simulink model "transfer_function_calculation"  (R2016a)
settings: Solver=VariableStepAuto  StartTime=0.0  StopTime=5  RelTol=1e-3
values from neighbouring files (symbols this model uses):
  a = .7    (= 0.7)    [PM_1_5MW_syn_27.m]
  Flux = 5.8264    [PM_1_5MW_syn_27.m]
  Id_set = 500    [PM_1_5MW_syn_27.m]
  Iq_set = -2200    [PM_1_5MW_syn_27.m]
  L = .0001    (= 0.0001)    [PM_1_5MW_syn_27.m]
  Ld = 0.001575    [PM_1_5MW_syn_27.m]
  Lq = 0.001575    [PM_1_5MW_syn_27.m]
  mn = 60000    [PM_1_5MW_syn_27.m]
  p = 26    [PM_1_5MW_syn_27.m]
  Rs = 0.000821    [PM_1_5MW_syn_27.m]
  Sollkurve_M_Optimum = [0 57121 101549 158670 228485 310994 406196 514092 634681 767965 810425 823386 ... (13 elements, 13x1)]    [Lookup_M_n.mat]
  Sollkurve_nGen_Optimum = [0 5 7 9 11 12 14 16 18 20 20.07 20.2 ... (13 elements, 13x1)]    [Lookup_M_n.mat]
  Speed_set = w_m    (= 2.10172548525)    [PM_1_5MW_syn_27.m]
  Ts_Power = 5.000000000000000e-06    (= 5e-06)    [PM_1_5MW_syn_27.m]
  Vdc = 1200    [PM_1_5MW_syn_27.m]
  Vh = Vm/6*0    (= 0)    [PM_1_5MW_syn_27.m]
undefined symbols (not defined in the file or in its folder): C2, Esw_Erec, Esw_Off, Esw_On, Page_Temp_C
undefined symbols (not defined in the file): Ts_Control, z
libraries: fl_lib x84, powerlib_meascontrol x58, simulink x56, nesl_utility x36, powerlib x33, simulink_extras x11
(part 6 of 6)

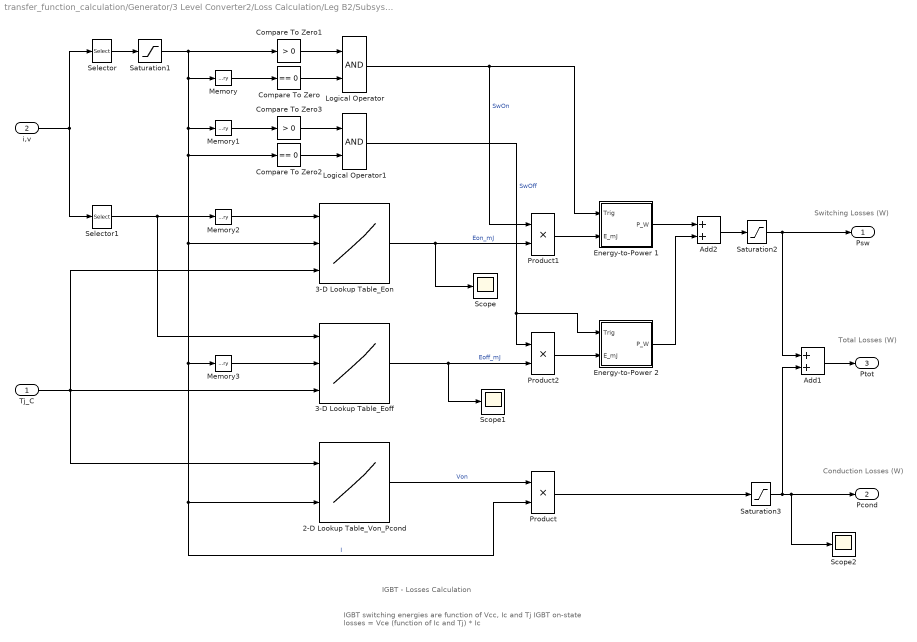
== system transfer_function_calculation/Generator/3 Level Converter2/Loss Calculation/Leg B2/Subsystem/Loss Calculation Unit/IGBTs Losses Calculation ==
  note: IGBT - Losses Calculation
  note: Switching Losses (W)
  note: Conduction Losses (W)
  note: Total Losses (W)
  note: IGBT switching energies are function of Vcc, Ic and Tj
      | IGBT on-state losses = Vce (function of Ic and Tj) * Ic
  Tj_C : Inport
  i,v : Inport  Port=2  PortDimensions=4
  2-D Lookup Table_Von_Pcond : Lookup_n-D  BreakpointsForDimension1=IGBT_Tj_OnState  BreakpointsForDimension2=IGBT_Ic_OnState  BreakpointsForDimension3=Page_Temp_C  Table=IGBT_Vce_OnState  RndMeth=Simplest  InputSameDT=on
  3-D Lookup Table_Eoff : Lookup_n-D  NumberOfTableDimensions=3  BreakpointsForDimension1=Vcc_Esw_Off  BreakpointsForDimension2=IGBT_Ic_Eoff  BreakpointsForDimension3=IGBT_Tj_Eoff  Table=Esw_Off  RndMeth=Simplest  InputSameDT=on
  3-D Lookup Table_Eon : Lookup_n-D  NumberOfTableDimensions=3  BreakpointsForDimension1=Vcc_Esw_On  BreakpointsForDimension2=IGBT_Ic_Eon  BreakpointsForDimension3=IGBT_Tj_Eon  Table=Esw_On  RndMeth=Simplest  InputSameDT=on
  Add1 : Sum
  Add2 : Sum
  Compare To Zero : simulink/Logic and Bit Operations/Compare To Zero  relop===  OutDataTypeStr=boolean
  Compare To Zero1 : simulink/Logic and Bit Operations/Compare To Zero  relop=>  OutDataTypeStr=boolean
  Compare To Zero2 : simulink/Logic and Bit Operations/Compare To Zero  relop===  OutDataTypeStr=boolean
  Compare To Zero3 : simulink/Logic and Bit Operations/Compare To Zero  relop=>  OutDataTypeStr=boolean
  Energy-to-Power 1 : Subsystem  mask{PulseDuration=PulseDuration, Ts=Ts}
      mask prompts: PulseDuration "Pulse Duration (s):"; Ts "Sample time (s):"
  Energy-to-Power 2 : Subsystem  mask{PulseDuration=PulseDuration, Ts=Ts}
      mask prompts: PulseDuration "Pulse Duration (s):"; Ts "Sample time (s):"
  Logical Operator : Logic  AllPortsSameDT=off  OutDataTypeStr=float('double')
  Logical Operator1 : Logic  AllPortsSameDT=off  OutDataTypeStr=float('double')
  Memory{,1..3} (4 alike) : Memory
  Product : Product  RndMeth=Zero
  Product1 : Product  RndMeth=Zero
  Product2 : Product  RndMeth=Zero
  Saturation1 : Saturate  UpperLimit=inf  LowerLimit=0
  Saturation2 : Saturate  UpperLimit=inf  LowerLimit=0
  Saturation3 : Saturate  UpperLimit=inf  LowerLimit=0
  Scope : Scope
  Scope1 : Scope
  Scope2 : Scope
  Selector : Selector  InputPortWidth=4  IndexOptions=Index vector (dialog)  Indices="[ 1  3 ]"  OutputSizes=1
  Selector1 : Selector  InputPortWidth=4  IndexOptions=Index vector (dialog)  Indices=[ 2 4 ]  OutputSizes=1
  Psw : Outport
  Pcond : Outport  Port=2
  Ptot : Outport  Port=3
  wires:
  Saturation3/1 -> Add1/2, Pcond/1, Scope2/1
  Saturation2/1 -> Add1/1, Psw/1
  Add2/1 -> Saturation2/1
  Memory1/1 -> Compare To Zero3/1
  Logical Operator1/1 -> Product2/1, Energy-to-Power 2/1(Trig)  "SwOff"
  Compare To Zero2/1 -> Logical Operator1/2
  Compare To Zero3/1 -> Logical Operator1/1
  Selector1/1 -> 3-D Lookup Table_Eoff/1, Memory2/1
  Logical Operator/1 -> Energy-to-Power 1/1(Trig), Product1/1  "SwOn"
  Compare To Zero/1 -> Logical Operator/2
  Compare To Zero1/1 -> Logical Operator/1
  Saturation1/1 -> Compare To Zero2/1, Product/2, 2-D Lookup Table_Von_Pcond/2, Memory3/1, 3-D Lookup Table_Eon/2, Memory1/1, Memory/1, Compare To Zero1/1  "I"
  Memory/1 -> Compare To Zero/1
  i,v/1 -> Selector/1, Selector1/1
  Add1/1 -> Ptot/1
  Selector/1 -> Saturation1/1
  Memory2/1 -> 3-D Lookup Table_Eon/1
  Memory3/1 -> 3-D Lookup Table_Eoff/2
  3-D Lookup Table_Eon/1 -> Product1/2, Scope/1  "Eon_mJ"
  3-D Lookup Table_Eoff/1 -> Product2/2, Scope1/1  "Eoff_mJ"
  Product/1 -> Saturation3/1
  Tj_C/1 -> 3-D Lookup Table_Eoff/3, 2-D Lookup Table_Von_Pcond/1, 3-D Lookup Table_Eon/3
  2-D Lookup Table_Von_Pcond/1 -> Product/1  "Von"
  Energy-to-Power 1/1(P_W) -> Add2/1
  Product1/1 -> Energy-to-Power 1/2(E_mJ)
  Product2/1 -> Energy-to-Power 2/2(E_mJ)
  Energy-to-Power 2/1(P_W) -> Add2/2

== system transfer_function_calculation/Generator/3 Level Converter2/Loss Calculation/Leg B2/Subsystem/Loss Calculation Unit/Thermal Model ==
  P_IGBTs : Inport  PortDimensions=2
  P_Diodes : Inport  Port=2  PortDimensions=2
  Tcase : Inport  Port=3  PortDimensions=1
  Add : Sum  Inputs=++++
  Demux{,1..5} (6 alike) : Demux  Outputs=2
  Discrete State-Space1 : DiscreteStateSpace  A=Ad_IGBT  B=Bd_IGBT  C=Cd_IGBT  D=Dd_IGBT  X0=x0d  SampleTime=Ts
  Discrete State-Space2 : DiscreteStateSpace  A=Ad_IGBT  B=Bd_IGBT  C=Cd_IGBT  D=Dd_IGBT  X0=x0d  SampleTime=Ts
  Discrete State-Space3 : DiscreteStateSpace  A=Ad_Diode  B=Bd_Diode  C=Cd_Diode  D=Dd_Diode  X0=x0d  SampleTime=Ts
  Discrete State-Space4 : DiscreteStateSpace  A=Ad_Diode  B=Bd_Diode  C=Cd_Diode  D=Dd_Diode  X0=x0d  SampleTime=Ts
  Memory1 : Memory
  Memory2 : Memory  X0=Tj0
  Memory3 : Memory  X0=Tj0
  Mux{,1..5} (6 alike) : Mux  Inputs=2
  Tj_IGBTs : Outport
  Pout : Outport  Port=2
  Tj_Diodes : Outport  Port=3
  wires:
  Mux3/1 -> Discrete State-Space4/1
  Mux2/1 -> Discrete State-Space3/1
  Mux1/1 -> Discrete State-Space2/1
  Mux/1 -> Discrete State-Space1/1
  Discrete State-Space1/1 -> Demux2/1
  Discrete State-Space2/1 -> Demux3/1
  Discrete State-Space3/1 -> Demux4/1
  Discrete State-Space4/1 -> Demux5/1
  Add/1 -> Memory1/1
  Demux1/1 -> Mux2/2
  Demux/1 -> Mux/2
  Demux/2 -> Mux1/2
  Demux1/2 -> Mux3/2
  Demux2/1 -> Mux4/1
  Demux3/1 -> Mux4/2
  Mux4/1 -> Memory2/1
  Demux4/1 -> Mux5/1
  Demux5/1 -> Mux5/2
  Demux2/2 -> Add/1
  Demux3/2 -> Add/2
  Demux4/2 -> Add/3
  Demux5/2 -> Add/4
  Mux5/1 -> Memory3/1
  P_IGBTs/1 -> Demux/1
  P_Diodes/1 -> Demux1/1
  Tcase/1 -> Mux3/1, Mux2/1, Mux/1, Mux1/1
  Memory1/1 -> Pout/1
  Memory3/1 -> Tj_Diodes/1
  Memory2/1 -> Tj_IGBTs/1

== system transfer_function_calculation/Generator/3 Level Converter2/Loss Calculation/Leg C1/Subsystem/Loss Calculation Unit/Demux IGBTs and Diodes Currents and voltages ==
  QD1 : Inport
  QD2 : Inport  Port=2
  Demux1 : Demux  Outputs=2
  Demux2 : Demux  Outputs=2
  Mux{1..6} (6 alike) : Mux  Inputs=2
  Scope : Scope
  Scope1 : Scope
  Subsystem1 : Subsystem
  Subsystem2 : Subsystem
  IGBTs : Outport
  Diodes : Outport  Port=2
  wires:
  Demux1/1 -> Subsystem1/1(I)
  Subsystem1/1(I_Q) -> Mux4/1
  Demux1/2 -> Mux1/2, Mux4/2
  Subsystem1/2(I_D) -> Mux1/1
  Demux2/1 -> Subsystem2/1(I)
  Subsystem2/1(I_Q) -> Mux3/1
  Demux2/2 -> Mux3/2, Mux2/2
  Subsystem2/2(I_D) -> Mux2/1
  Mux4/1 -> Scope/1, Mux5/1
  Mux3/1 -> Mux5/2
  Mux1/1 -> Scope1/1, Mux6/1
  Mux2/1 -> Mux6/2
  QD1/1 -> Demux1/1
  Mux5/1 -> IGBTs/1
  QD2/1 -> Demux2/1
  Mux6/1 -> Diodes/1

== system transfer_function_calculation/Generator/3 Level Converter2/Loss Calculation/Leg C1/Subsystem/Loss Calculation Unit/Diodes Losses Calculation ==
  note: Conduction Losses (W)
  note: Total Losses (W)
  note: Reverse Recovery Losses (W)
  note: Reverse recovery energy (Erec)is function of Vcc, If and Tj
      | Diode on-state losses = Vf (function of If and Tj) * If
  note: Diode - Losses Calculation
  i,v : Inport  PortDimensions=4
  Tj_C : Inport  Port=2
  2-D Lookup Table_Vf_on_Diode_Pcond : Lookup_n-D  BreakpointsForDimension1=DIODE_Tj_OnState  BreakpointsForDimension2=DIODE_If_OnState  BreakpointsForDimension3=Page_Temp_C  Table=DIODE_Vf_OnState  RndMeth=Simplest  InputSameDT=on
  3-D Lookup Table_Erec_Diode : Lookup_n-D  NumberOfTableDimensions=3  BreakpointsForDimension1=Vcc_Esw_Erec  BreakpointsForDimension2=DIODE_If_Erec  BreakpointsForDimension3=DIODE_Tj_Erec  Table=Esw_Erec  RndMeth=Simplest  InputSameDT=on
  Add1 : Sum
  Compare To Zero : simulink/Logic and Bit Operations/Compare To Zero  relop===  OutDataTypeStr=boolean
  Compare To Zero1 : simulink/Logic and Bit Operations/Compare To Zero  relop=>  OutDataTypeStr=boolean
  Energy-to-Power 2 : Subsystem  mask{PulseDuration=PulseDuration, Ts=Ts}
      mask prompts: PulseDuration "Pulse Duration (s):"; Ts "Sample time (s):"
  Logical Operator : Logic  AllPortsSameDT=off  OutDataTypeStr=float('double')
  Memory2 : Memory
  Product : Product  RndMeth=Zero
  Product1 : Product  RndMeth=Zero
  Saturation1 : Saturate  UpperLimit=inf  LowerLimit=0
  Saturation2 : Saturate  UpperLimit=inf  LowerLimit=0
  Selector2 : Selector  InputPortWidth=4  IndexOptions=Index vector (dialog)  Indices="[ 1  3 ]"  OutputSizes=1
  Selector3 : Selector  InputPortWidth=4  IndexOptions=Index vector (dialog)  Indices=[ 2 4 ]  OutputSizes=1
  Ptot : Outport
  Psw : Outport  Port=2
  Pcond : Outport  Port=3
  wires:
  Energy-to-Power 2/1(P_W) -> Saturation2/1
  Product1/1 -> Energy-to-Power 2/2(E_mJ)
  Product/1 -> Saturation1/1
  Tj_C/1 -> 2-D Lookup Table_Vf_on_Diode_Pcond/1, 3-D Lookup Table_Erec_Diode/3
  2-D Lookup Table_Vf_on_Diode_Pcond/1 -> Product/1  "Vf_on_Diode"
  Add1/1 -> Ptot/1
  Compare To Zero1/1 -> Logical Operator/1
  Compare To Zero/1 -> Logical Operator/2
  Logical Operator/1 -> Energy-to-Power 2/1(Trig), Product1/1
  3-D Lookup Table_Erec_Diode/1 -> Product1/2  "Erec_mJ"
  Selector2/1 -> Memory2/1, Compare To Zero/1, 2-D Lookup Table_Vf_on_Diode_Pcond/2, Product/2  "If"
  i,v/1 -> Selector2/1, Selector3/1
  Selector3/1 -> 3-D Lookup Table_Erec_Diode/1
  Memory2/1 -> Compare To Zero1/1, 3-D Lookup Table_Erec_Diode/2
  Saturation2/1 -> Psw/1, Add1/1
  Saturation1/1 -> Add1/2, Pcond/1

== system transfer_function_calculation/Generator/3 Level Converter2/Loss Calculation/Leg C1/Subsystem/Loss Calculation Unit/IGBTs Losses Calculation ==
  note: IGBT switching energies are function of Vcc, Ic and Tj
      | IGBT on-state losses = Vce (function of Ic and Tj) * Ic
  note: Total Losses (W)
  note: Conduction Losses (W)
  note: Switching Losses (W)
  note: IGBT - Losses Calculation
  Tj_C : Inport
  i,v : Inport  Port=2  PortDimensions=4
  2-D Lookup Table_Von_Pcond : Lookup_n-D  BreakpointsForDimension1=IGBT_Tj_OnState  BreakpointsForDimension2=IGBT_Ic_OnState  BreakpointsForDimension3=Page_Temp_C  Table=IGBT_Vce_OnState  RndMeth=Simplest  InputSameDT=on
  3-D Lookup Table_Eoff : Lookup_n-D  NumberOfTableDimensions=3  BreakpointsForDimension1=Vcc_Esw_Off  BreakpointsForDimension2=IGBT_Ic_Eoff  BreakpointsForDimension3=IGBT_Tj_Eoff  Table=Esw_Off  RndMeth=Simplest  InputSameDT=on
  3-D Lookup Table_Eon : Lookup_n-D  NumberOfTableDimensions=3  BreakpointsForDimension1=Vcc_Esw_On  BreakpointsForDimension2=IGBT_Ic_Eon  BreakpointsForDimension3=IGBT_Tj_Eon  Table=Esw_On  RndMeth=Simplest  InputSameDT=on
  Add1 : Sum
  Add2 : Sum
  Compare To Zero : simulink/Logic and Bit Operations/Compare To Zero  relop===  OutDataTypeStr=boolean
  Compare To Zero1 : simulink/Logic and Bit Operations/Compare To Zero  relop=>  OutDataTypeStr=boolean
  Compare To Zero2 : simulink/Logic and Bit Operations/Compare To Zero  relop===  OutDataTypeStr=boolean
  Compare To Zero3 : simulink/Logic and Bit Operations/Compare To Zero  relop=>  OutDataTypeStr=boolean
  Energy-to-Power 1 : Subsystem  mask{PulseDuration=PulseDuration, Ts=Ts}
      mask prompts: PulseDuration "Pulse Duration (s):"; Ts "Sample time (s):"
  Energy-to-Power 2 : Subsystem  mask{PulseDuration=PulseDuration, Ts=Ts}
      mask prompts: PulseDuration "Pulse Duration (s):"; Ts "Sample time (s):"
  Logical Operator : Logic  AllPortsSameDT=off  OutDataTypeStr=float('double')
  Logical Operator1 : Logic  AllPortsSameDT=off  OutDataTypeStr=float('double')
  Memory{,1..3} (4 alike) : Memory
  Product : Product  RndMeth=Zero
  Product1 : Product  RndMeth=Zero
  Product2 : Product  RndMeth=Zero
  Saturation1 : Saturate  UpperLimit=inf  LowerLimit=0
  Saturation2 : Saturate  UpperLimit=inf  LowerLimit=0
  Saturation3 : Saturate  UpperLimit=inf  LowerLimit=0
  Scope : Scope
  Scope1 : Scope
  Scope2 : Scope
  Selector : Selector  InputPortWidth=4  IndexOptions=Index vector (dialog)  Indices="[ 1  3 ]"  OutputSizes=1
  Selector1 : Selector  InputPortWidth=4  IndexOptions=Index vector (dialog)  Indices=[ 2 4 ]  OutputSizes=1
  Psw : Outport
  Pcond : Outport  Port=2
  Ptot : Outport  Port=3
  wires:
  Energy-to-Power 2/1(P_W) -> Add2/2
  Product2/1 -> Energy-to-Power 2/2(E_mJ)
  Product1/1 -> Energy-to-Power 1/2(E_mJ)
  Energy-to-Power 1/1(P_W) -> Add2/1
  2-D Lookup Table_Von_Pcond/1 -> Product/1  "Von"
  Tj_C/1 -> 3-D Lookup Table_Eon/3, 2-D Lookup Table_Von_Pcond/1, 3-D Lookup Table_Eoff/3
  Product/1 -> Saturation3/1
  3-D Lookup Table_Eoff/1 -> Scope1/1, Product2/2  "Eoff_mJ"
  3-D Lookup Table_Eon/1 -> Scope/1, Product1/2  "Eon_mJ"
  Memory3/1 -> 3-D Lookup Table_Eoff/2
  Memory2/1 -> 3-D Lookup Table_Eon/1
  Selector/1 -> Saturation1/1
  Add1/1 -> Ptot/1
  i,v/1 -> Selector1/1, Selector/1
  Memory/1 -> Compare To Zero/1
  Saturation1/1 -> Compare To Zero1/1, Memory/1, Memory1/1, 3-D Lookup Table_Eon/2, Memory3/1, 2-D Lookup Table_Von_Pcond/2, Product/2, Compare To Zero2/1  "I"
  Compare To Zero1/1 -> Logical Operator/1
  Compare To Zero/1 -> Logical Operator/2
  Logical Operator/1 -> Product1/1, Energy-to-Power 1/1(Trig)  "SwOn"
  Selector1/1 -> Memory2/1, 3-D Lookup Table_Eoff/1
  Compare To Zero3/1 -> Logical Operator1/1
  Compare To Zero2/1 -> Logical Operator1/2
  Logical Operator1/1 -> Energy-to-Power 2/1(Trig), Product2/1  "SwOff"
  Memory1/1 -> Compare To Zero3/1
  Add2/1 -> Saturation2/1
  Saturation2/1 -> Psw/1, Add1/1
  Saturation3/1 -> Scope2/1, Pcond/1, Add1/2

== system transfer_function_calculation/Generator/3 Level Converter2/Loss Calculation/Leg C1/Subsystem/Loss Calculation Unit/Thermal Model ==
  P_IGBTs : Inport  PortDimensions=2
  P_Diodes : Inport  Port=2  PortDimensions=2
  Tcase : Inport  Port=3  PortDimensions=1
  Add : Sum  Inputs=++++
  Demux{,1..5} (6 alike) : Demux  Outputs=2
  Discrete State-Space1 : DiscreteStateSpace  A=Ad_IGBT  B=Bd_IGBT  C=Cd_IGBT  D=Dd_IGBT  X0=x0d  SampleTime=Ts
  Discrete State-Space2 : DiscreteStateSpace  A=Ad_IGBT  B=Bd_IGBT  C=Cd_IGBT  D=Dd_IGBT  X0=x0d  SampleTime=Ts
  Discrete State-Space3 : DiscreteStateSpace  A=Ad_Diode  B=Bd_Diode  C=Cd_Diode  D=Dd_Diode  X0=x0d  SampleTime=Ts
  Discrete State-Space4 : DiscreteStateSpace  A=Ad_Diode  B=Bd_Diode  C=Cd_Diode  D=Dd_Diode  X0=x0d  SampleTime=Ts
  Memory1 : Memory
  Memory2 : Memory  X0=Tj0
  Memory3 : Memory  X0=Tj0
  Mux{,1..5} (6 alike) : Mux  Inputs=2
  Tj_IGBTs : Outport
  Pout : Outport  Port=2
  Tj_Diodes : Outport  Port=3
  wires:
  Memory2/1 -> Tj_IGBTs/1
  Memory3/1 -> Tj_Diodes/1
  Memory1/1 -> Pout/1
  Tcase/1 -> Mux1/1, Mux/1, Mux2/1, Mux3/1
  P_Diodes/1 -> Demux1/1
  P_IGBTs/1 -> Demux/1
  Mux5/1 -> Memory3/1
  Demux5/2 -> Add/4
  Demux4/2 -> Add/3
  Demux3/2 -> Add/2
  Demux2/2 -> Add/1
  Demux5/1 -> Mux5/2
  Demux4/1 -> Mux5/1
  Mux4/1 -> Memory2/1
  Demux3/1 -> Mux4/2
  Demux2/1 -> Mux4/1
  Demux1/2 -> Mux3/2
  Demux/2 -> Mux1/2
  Demux/1 -> Mux/2
  Demux1/1 -> Mux2/2
  Add/1 -> Memory1/1
  Discrete State-Space4/1 -> Demux5/1
  Discrete State-Space3/1 -> Demux4/1
  Discrete State-Space2/1 -> Demux3/1
  Discrete State-Space1/1 -> Demux2/1
  Mux/1 -> Discrete State-Space1/1
  Mux1/1 -> Discrete State-Space2/1
  Mux2/1 -> Discrete State-Space3/1
  Mux3/1 -> Discrete State-Space4/1

== system transfer_function_calculation/Generator/3 Level Converter2/Loss Calculation/Leg C2/Subsystem/Loss Calculation Unit/Demux IGBTs and Diodes Currents and voltages ==
  QD1 : Inport
  QD2 : Inport  Port=2
  Demux1 : Demux  Outputs=2
  Demux2 : Demux  Outputs=2
  Mux{1..6} (6 alike) : Mux  Inputs=2
  Scope : Scope
  Scope1 : Scope
  Subsystem1 : Subsystem
  Subsystem2 : Subsystem
  IGBTs : Outport
  Diodes : Outport  Port=2
  wires:
  Mux6/1 -> Diodes/1
  QD2/1 -> Demux2/1
  Mux5/1 -> IGBTs/1
  QD1/1 -> Demux1/1
  Mux2/1 -> Mux6/2
  Mux1/1 -> Mux6/1, Scope1/1
  Mux3/1 -> Mux5/2
  Mux4/1 -> Mux5/1, Scope/1
  Subsystem2/2(I_D) -> Mux2/1
  Demux2/2 -> Mux2/2, Mux3/2
  Subsystem2/1(I_Q) -> Mux3/1
  Demux2/1 -> Subsystem2/1(I)
  Subsystem1/2(I_D) -> Mux1/1
  Demux1/2 -> Mux4/2, Mux1/2
  Subsystem1/1(I_Q) -> Mux4/1
  Demux1/1 -> Subsystem1/1(I)

== system transfer_function_calculation/Generator/3 Level Converter2/Loss Calculation/Leg C2/Subsystem/Loss Calculation Unit/Diodes Losses Calculation ==
  note: Diode - Losses Calculation
  note: Reverse recovery energy (Erec)is function of Vcc, If and Tj
      | Diode on-state losses = Vf (function of If and Tj) * If
  note: Reverse Recovery Losses (W)
  note: Total Losses (W)
  note: Conduction Losses (W)
  i,v : Inport  PortDimensions=4
  Tj_C : Inport  Port=2
  2-D Lookup Table_Vf_on_Diode_Pcond : Lookup_n-D  BreakpointsForDimension1=DIODE_Tj_OnState  BreakpointsForDimension2=DIODE_If_OnState  BreakpointsForDimension3=Page_Temp_C  Table=DIODE_Vf_OnState  RndMeth=Simplest  InputSameDT=on
  3-D Lookup Table_Erec_Diode : Lookup_n-D  NumberOfTableDimensions=3  BreakpointsForDimension1=Vcc_Esw_Erec  BreakpointsForDimension2=DIODE_If_Erec  BreakpointsForDimension3=DIODE_Tj_Erec  Table=Esw_Erec  RndMeth=Simplest  InputSameDT=on
  Add1 : Sum
  Compare To Zero : simulink/Logic and Bit Operations/Compare To Zero  relop===  OutDataTypeStr=boolean
  Compare To Zero1 : simulink/Logic and Bit Operations/Compare To Zero  relop=>  OutDataTypeStr=boolean
  Energy-to-Power 2 : Subsystem  mask{PulseDuration=PulseDuration, Ts=Ts}
      mask prompts: PulseDuration "Pulse Duration (s):"; Ts "Sample time (s):"
  Logical Operator : Logic  AllPortsSameDT=off  OutDataTypeStr=float('double')
  Memory2 : Memory
  Product : Product  RndMeth=Zero
  Product1 : Product  RndMeth=Zero
  Saturation1 : Saturate  UpperLimit=inf  LowerLimit=0
  Saturation2 : Saturate  UpperLimit=inf  LowerLimit=0
  Selector2 : Selector  InputPortWidth=4  IndexOptions=Index vector (dialog)  Indices="[ 1  3 ]"  OutputSizes=1
  Selector3 : Selector  InputPortWidth=4  IndexOptions=Index vector (dialog)  Indices=[ 2 4 ]  OutputSizes=1
  Ptot : Outport
  Psw : Outport  Port=2
  Pcond : Outport  Port=3
  wires:
  Saturation1/1 -> Pcond/1, Add1/2
  Saturation2/1 -> Add1/1, Psw/1
  Memory2/1 -> 3-D Lookup Table_Erec_Diode/2, Compare To Zero1/1
  Selector3/1 -> 3-D Lookup Table_Erec_Diode/1
  i,v/1 -> Selector3/1, Selector2/1
  Selector2/1 -> Product/2, 2-D Lookup Table_Vf_on_Diode_Pcond/2, Compare To Zero/1, Memory2/1  "If"
  3-D Lookup Table_Erec_Diode/1 -> Product1/2  "Erec_mJ"
  Logical Operator/1 -> Product1/1, Energy-to-Power 2/1(Trig)
  Compare To Zero/1 -> Logical Operator/2
  Compare To Zero1/1 -> Logical Operator/1
  Add1/1 -> Ptot/1
  2-D Lookup Table_Vf_on_Diode_Pcond/1 -> Product/1  "Vf_on_Diode"
  Tj_C/1 -> 3-D Lookup Table_Erec_Diode/3, 2-D Lookup Table_Vf_on_Diode_Pcond/1
  Product/1 -> Saturation1/1
  Product1/1 -> Energy-to-Power 2/2(E_mJ)
  Energy-to-Power 2/1(P_W) -> Saturation2/1

== system transfer_function_calculation/Generator/3 Level Converter2/Loss Calculation/Leg C2/Subsystem/Loss Calculation Unit/IGBTs Losses Calculation ==
  note: IGBT - Losses Calculation
  note: Switching Losses (W)
  note: Conduction Losses (W)
  note: Total Losses (W)
  note: IGBT switching energies are function of Vcc, Ic and Tj
      | IGBT on-state losses = Vce (function of Ic and Tj) * Ic
  Tj_C : Inport
  i,v : Inport  Port=2  PortDimensions=4
  2-D Lookup Table_Von_Pcond : Lookup_n-D  BreakpointsForDimension1=IGBT_Tj_OnState  BreakpointsForDimension2=IGBT_Ic_OnState  BreakpointsForDimension3=Page_Temp_C  Table=IGBT_Vce_OnState  RndMeth=Simplest  InputSameDT=on
  3-D Lookup Table_Eoff : Lookup_n-D  NumberOfTableDimensions=3  BreakpointsForDimension1=Vcc_Esw_Off  BreakpointsForDimension2=IGBT_Ic_Eoff  BreakpointsForDimension3=IGBT_Tj_Eoff  Table=Esw_Off  RndMeth=Simplest  InputSameDT=on
  3-D Lookup Table_Eon : Lookup_n-D  NumberOfTableDimensions=3  BreakpointsForDimension1=Vcc_Esw_On  BreakpointsForDimension2=IGBT_Ic_Eon  BreakpointsForDimension3=IGBT_Tj_Eon  Table=Esw_On  RndMeth=Simplest  InputSameDT=on
  Add1 : Sum
  Add2 : Sum
  Compare To Zero : simulink/Logic and Bit Operations/Compare To Zero  relop===  OutDataTypeStr=boolean
  Compare To Zero1 : simulink/Logic and Bit Operations/Compare To Zero  relop=>  OutDataTypeStr=boolean
  Compare To Zero2 : simulink/Logic and Bit Operations/Compare To Zero  relop===  OutDataTypeStr=boolean
  Compare To Zero3 : simulink/Logic and Bit Operations/Compare To Zero  relop=>  OutDataTypeStr=boolean
  Energy-to-Power 1 : Subsystem  mask{PulseDuration=PulseDuration, Ts=Ts}
      mask prompts: PulseDuration "Pulse Duration (s):"; Ts "Sample time (s):"
  Energy-to-Power 2 : Subsystem  mask{PulseDuration=PulseDuration, Ts=Ts}
      mask prompts: PulseDuration "Pulse Duration (s):"; Ts "Sample time (s):"
  Logical Operator : Logic  AllPortsSameDT=off  OutDataTypeStr=float('double')
  Logical Operator1 : Logic  AllPortsSameDT=off  OutDataTypeStr=float('double')
  Memory{,1..3} (4 alike) : Memory
  Product : Product  RndMeth=Zero
  Product1 : Product  RndMeth=Zero
  Product2 : Product  RndMeth=Zero
  Saturation1 : Saturate  UpperLimit=inf  LowerLimit=0
  Saturation2 : Saturate  UpperLimit=inf  LowerLimit=0
  Saturation3 : Saturate  UpperLimit=inf  LowerLimit=0
  Scope : Scope
  Scope1 : Scope
  Scope2 : Scope
  Selector : Selector  InputPortWidth=4  IndexOptions=Index vector (dialog)  Indices="[ 1  3 ]"  OutputSizes=1
  Selector1 : Selector  InputPortWidth=4  IndexOptions=Index vector (dialog)  Indices=[ 2 4 ]  OutputSizes=1
  Psw : Outport
  Pcond : Outport  Port=2
  Ptot : Outport  Port=3
  wires:
  Saturation3/1 -> Add1/2, Pcond/1, Scope2/1
  Saturation2/1 -> Add1/1, Psw/1
  Add2/1 -> Saturation2/1
  Memory1/1 -> Compare To Zero3/1
  Logical Operator1/1 -> Product2/1, Energy-to-Power 2/1(Trig)  "SwOff"
  Compare To Zero2/1 -> Logical Operator1/2
  Compare To Zero3/1 -> Logical Operator1/1
  Selector1/1 -> 3-D Lookup Table_Eoff/1, Memory2/1
  Logical Operator/1 -> Energy-to-Power 1/1(Trig), Product1/1  "SwOn"
  Compare To Zero/1 -> Logical Operator/2
  Compare To Zero1/1 -> Logical Operator/1
  Saturation1/1 -> Compare To Zero2/1, Product/2, 2-D Lookup Table_Von_Pcond/2, Memory3/1, 3-D Lookup Table_Eon/2, Memory1/1, Memory/1, Compare To Zero1/1  "I"
  Memory/1 -> Compare To Zero/1
  i,v/1 -> Selector/1, Selector1/1
  Add1/1 -> Ptot/1
  Selector/1 -> Saturation1/1
  Memory2/1 -> 3-D Lookup Table_Eon/1
  Memory3/1 -> 3-D Lookup Table_Eoff/2
  3-D Lookup Table_Eon/1 -> Product1/2, Scope/1  "Eon_mJ"
  3-D Lookup Table_Eoff/1 -> Product2/2, Scope1/1  "Eoff_mJ"
  Product/1 -> Saturation3/1
  Tj_C/1 -> 3-D Lookup Table_Eoff/3, 2-D Lookup Table_Von_Pcond/1, 3-D Lookup Table_Eon/3
  2-D Lookup Table_Von_Pcond/1 -> Product/1  "Von"
  Energy-to-Power 1/1(P_W) -> Add2/1
  Product1/1 -> Energy-to-Power 1/2(E_mJ)
  Product2/1 -> Energy-to-Power 2/2(E_mJ)
  Energy-to-Power 2/1(P_W) -> Add2/2

== system transfer_function_calculation/Generator/3 Level Converter2/Loss Calculation/Leg C2/Subsystem/Loss Calculation Unit/Thermal Model ==
  P_IGBTs : Inport  PortDimensions=2
  P_Diodes : Inport  Port=2  PortDimensions=2
  Tcase : Inport  Port=3  PortDimensions=1
  Add : Sum  Inputs=++++
  Demux{,1..5} (6 alike) : Demux  Outputs=2
  Discrete State-Space1 : DiscreteStateSpace  A=Ad_IGBT  B=Bd_IGBT  C=Cd_IGBT  D=Dd_IGBT  X0=x0d  SampleTime=Ts
  Discrete State-Space2 : DiscreteStateSpace  A=Ad_IGBT  B=Bd_IGBT  C=Cd_IGBT  D=Dd_IGBT  X0=x0d  SampleTime=Ts
  Discrete State-Space3 : DiscreteStateSpace  A=Ad_Diode  B=Bd_Diode  C=Cd_Diode  D=Dd_Diode  X0=x0d  SampleTime=Ts
  Discrete State-Space4 : DiscreteStateSpace  A=Ad_Diode  B=Bd_Diode  C=Cd_Diode  D=Dd_Diode  X0=x0d  SampleTime=Ts
  Memory1 : Memory
  Memory2 : Memory  X0=Tj0
  Memory3 : Memory  X0=Tj0
  Mux{,1..5} (6 alike) : Mux  Inputs=2
  Tj_IGBTs : Outport
  Pout : Outport  Port=2
  Tj_Diodes : Outport  Port=3
  wires:
  Mux3/1 -> Discrete State-Space4/1
  Mux2/1 -> Discrete State-Space3/1
  Mux1/1 -> Discrete State-Space2/1
  Mux/1 -> Discrete State-Space1/1
  Discrete State-Space1/1 -> Demux2/1
  Discrete State-Space2/1 -> Demux3/1
  Discrete State-Space3/1 -> Demux4/1
  Discrete State-Space4/1 -> Demux5/1
  Add/1 -> Memory1/1
  Demux1/1 -> Mux2/2
  Demux/1 -> Mux/2
  Demux/2 -> Mux1/2
  Demux1/2 -> Mux3/2
  Demux2/1 -> Mux4/1
  Demux3/1 -> Mux4/2
  Mux4/1 -> Memory2/1
  Demux4/1 -> Mux5/1
  Demux5/1 -> Mux5/2
  Demux2/2 -> Add/1
  Demux3/2 -> Add/2
  Demux4/2 -> Add/3
  Demux5/2 -> Add/4
  Mux5/1 -> Memory3/1
  P_IGBTs/1 -> Demux/1
  P_Diodes/1 -> Demux1/1
  Tcase/1 -> Mux3/1, Mux2/1, Mux/1, Mux1/1
  Memory1/1 -> Pout/1
  Memory3/1 -> Tj_Diodes/1
  Memory2/1 -> Tj_IGBTs/1

== system transfer_function_calculation/Generator/3 Level Converter2/Loss Calculation/Leg A1/Subsystem/Loss Calculation Unit/Demux IGBTs and Diodes Currents and voltages/Subsystem1 ==
  I : Inport
  Gain1 : Gain  Gain=-1
  Saturation2 : Saturate  UpperLimit=1e6  LowerLimit=0
  Saturation3 : Saturate  UpperLimit=0  LowerLimit=-1e6
  I_Q : Outport
  I_D : Outport  Port=2
  wires:
  Gain1/1 -> I_D/1
  Saturation2/1 -> I_Q/1
  I/1 -> Saturation3/1, Saturation2/1
  Saturation3/1 -> Gain1/1

== system transfer_function_calculation/Generator/3 Level Converter2/Loss Calculation/Leg A1/Subsystem/Loss Calculation Unit/Demux IGBTs and Diodes Currents and voltages/Subsystem2 ==
  I : Inport
  Gain1 : Gain  Gain=-1
  Saturation2 : Saturate  UpperLimit=1e6  LowerLimit=0
  Saturation3 : Saturate  UpperLimit=0  LowerLimit=-1e6
  I_Q : Outport
  I_D : Outport  Port=2
  wires:
  Saturation3/1 -> Gain1/1
  I/1 -> Saturation2/1, Saturation3/1
  Saturation2/1 -> I_Q/1
  Gain1/1 -> I_D/1

== system transfer_function_calculation/Generator/3 Level Converter2/Loss Calculation/Leg A1/Subsystem/Loss Calculation Unit/Diodes Losses Calculation/Energy-to-Power 2 ==
  Trig : Inport
  E_mJ : Inport  Port=2
  Constant2 : Constant
  Constant3 : Constant  Value=0
  Monostable : powerlib_meascontrol/Logic/Monostable  EdgeDetect=Rising  PulseDuration=ceil(PulseDuration/Ts)*Ts  ic=0  Ts=Ts
  Product1 : Product  RndMeth=Zero
  Sample and Hold : powerlib_meascontrol/Additional Components/Sample and Hold  ic=0  Ts=Ts
  Switch1 : Switch  Criteria=u2 ~= 0
  gain : Gain  Gain=1e-3/(ceil(PulseDuration/Ts)*Ts)
  P_W : Outport
  wires:
  Switch1/1 -> Product1/2
  Constant3/1 -> Switch1/3
  Constant2/1 -> Switch1/1
  Monostable/1 -> Switch1/2
  E_mJ/1 -> gain/1
  Trig/1 -> Monostable/1, Sample and Hold/2
  gain/1 -> Sample and Hold/1
  Sample and Hold/1 -> Product1/1
  Product1/1 -> P_W/1

== system transfer_function_calculation/Generator/3 Level Converter2/Loss Calculation/Leg A1/Subsystem/Loss Calculation Unit/IGBTs Losses Calculation/Energy-to-Power 1 ==
  Trig : Inport
  E_mJ : Inport  Port=2
  Constant2 : Constant
  Constant3 : Constant  Value=0
  Monostable : powerlib_meascontrol/Logic/Monostable  EdgeDetect=Rising  PulseDuration=ceil(PulseDuration/Ts)*Ts  ic=0  Ts=Ts
  Product1 : Product  RndMeth=Zero
  Sample and Hold : powerlib_meascontrol/Additional Components/Sample and Hold  ic=0  Ts=Ts
  Switch1 : Switch  Criteria=u2 ~= 0
  gain : Gain  Gain=1e-3/(ceil(PulseDuration/Ts)*Ts)
  P_W : Outport
  wires:
  Switch1/1 -> Product1/2
  Constant3/1 -> Switch1/3
  Constant2/1 -> Switch1/1
  Monostable/1 -> Switch1/2
  E_mJ/1 -> gain/1
  Trig/1 -> Monostable/1, Sample and Hold/2
  gain/1 -> Sample and Hold/1
  Sample and Hold/1 -> Product1/1
  Product1/1 -> P_W/1

== system transfer_function_calculation/Generator/3 Level Converter2/Loss Calculation/Leg A1/Subsystem/Loss Calculation Unit/IGBTs Losses Calculation/Energy-to-Power 2 ==
  Trig : Inport
  E_mJ : Inport  Port=2
  Constant2 : Constant
  Constant3 : Constant  Value=0
  Monostable : powerlib_meascontrol/Logic/Monostable  EdgeDetect=Rising  PulseDuration=ceil(PulseDuration/Ts)*Ts  ic=0  Ts=Ts
  Product1 : Product  RndMeth=Zero
  Sample and Hold : powerlib_meascontrol/Additional Components/Sample and Hold  ic=0  Ts=Ts
  Switch1 : Switch  Criteria=u2 ~= 0
  gain : Gain  Gain=1e-3/(ceil(PulseDuration/Ts)*Ts)
  P_W : Outport
  wires:
  Switch1/1 -> Product1/2
  Constant3/1 -> Switch1/3
  Constant2/1 -> Switch1/1
  Monostable/1 -> Switch1/2
  E_mJ/1 -> gain/1
  Trig/1 -> Monostable/1, Sample and Hold/2
  gain/1 -> Sample and Hold/1
  Sample and Hold/1 -> Product1/1
  Product1/1 -> P_W/1

== system transfer_function_calculation/Generator/3 Level Converter2/Loss Calculation/Leg A2/Subsystem/Loss Calculation Unit/Demux IGBTs and Diodes Currents and voltages/Subsystem1 ==
  I : Inport
  Gain1 : Gain  Gain=-1
  Saturation2 : Saturate  UpperLimit=1e6  LowerLimit=0
  Saturation3 : Saturate  UpperLimit=0  LowerLimit=-1e6
  I_Q : Outport
  I_D : Outport  Port=2
  wires:
  Saturation3/1 -> Gain1/1
  I/1 -> Saturation2/1, Saturation3/1
  Saturation2/1 -> I_Q/1
  Gain1/1 -> I_D/1

== system transfer_function_calculation/Generator/3 Level Converter2/Loss Calculation/Leg A2/Subsystem/Loss Calculation Unit/Demux IGBTs and Diodes Currents and voltages/Subsystem2 ==
  I : Inport
  Gain1 : Gain  Gain=-1
  Saturation2 : Saturate  UpperLimit=1e6  LowerLimit=0
  Saturation3 : Saturate  UpperLimit=0  LowerLimit=-1e6
  I_Q : Outport
  I_D : Outport  Port=2
  wires:
  Gain1/1 -> I_D/1
  Saturation2/1 -> I_Q/1
  I/1 -> Saturation3/1, Saturation2/1
  Saturation3/1 -> Gain1/1

== system transfer_function_calculation/Generator/3 Level Converter2/Loss Calculation/Leg A2/Subsystem/Loss Calculation Unit/Diodes Losses Calculation/Energy-to-Power 2 ==
  Trig : Inport
  E_mJ : Inport  Port=2
  Constant2 : Constant
  Constant3 : Constant  Value=0
  Monostable : powerlib_meascontrol/Logic/Monostable  EdgeDetect=Rising  PulseDuration=ceil(PulseDuration/Ts)*Ts  ic=0  Ts=Ts
  Product1 : Product  RndMeth=Zero
  Sample and Hold : powerlib_meascontrol/Additional Components/Sample and Hold  ic=0  Ts=Ts
  Switch1 : Switch  Criteria=u2 ~= 0
  gain : Gain  Gain=1e-3/(ceil(PulseDuration/Ts)*Ts)
  P_W : Outport
  wires:
  Product1/1 -> P_W/1
  Sample and Hold/1 -> Product1/1
  gain/1 -> Sample and Hold/1
  Trig/1 -> Sample and Hold/2, Monostable/1
  E_mJ/1 -> gain/1
  Monostable/1 -> Switch1/2
  Constant2/1 -> Switch1/1
  Constant3/1 -> Switch1/3
  Switch1/1 -> Product1/2

== system transfer_function_calculation/Generator/3 Level Converter2/Loss Calculation/Leg A2/Subsystem/Loss Calculation Unit/IGBTs Losses Calculation/Energy-to-Power 1 ==
  Trig : Inport
  E_mJ : Inport  Port=2
  Constant2 : Constant
  Constant3 : Constant  Value=0
  Monostable : powerlib_meascontrol/Logic/Monostable  EdgeDetect=Rising  PulseDuration=ceil(PulseDuration/Ts)*Ts  ic=0  Ts=Ts
  Product1 : Product  RndMeth=Zero
  Sample and Hold : powerlib_meascontrol/Additional Components/Sample and Hold  ic=0  Ts=Ts
  Switch1 : Switch  Criteria=u2 ~= 0
  gain : Gain  Gain=1e-3/(ceil(PulseDuration/Ts)*Ts)
  P_W : Outport
  wires:
  Product1/1 -> P_W/1
  Sample and Hold/1 -> Product1/1
  gain/1 -> Sample and Hold/1
  Trig/1 -> Sample and Hold/2, Monostable/1
  E_mJ/1 -> gain/1
  Monostable/1 -> Switch1/2
  Constant2/1 -> Switch1/1
  Constant3/1 -> Switch1/3
  Switch1/1 -> Product1/2

== system transfer_function_calculation/Generator/3 Level Converter2/Loss Calculation/Leg A2/Subsystem/Loss Calculation Unit/IGBTs Losses Calculation/Energy-to-Power 2 ==
  Trig : Inport
  E_mJ : Inport  Port=2
  Constant2 : Constant
  Constant3 : Constant  Value=0
  Monostable : powerlib_meascontrol/Logic/Monostable  EdgeDetect=Rising  PulseDuration=ceil(PulseDuration/Ts)*Ts  ic=0  Ts=Ts
  Product1 : Product  RndMeth=Zero
  Sample and Hold : powerlib_meascontrol/Additional Components/Sample and Hold  ic=0  Ts=Ts
  Switch1 : Switch  Criteria=u2 ~= 0
  gain : Gain  Gain=1e-3/(ceil(PulseDuration/Ts)*Ts)
  P_W : Outport
  wires:
  Product1/1 -> P_W/1
  Sample and Hold/1 -> Product1/1
  gain/1 -> Sample and Hold/1
  Trig/1 -> Sample and Hold/2, Monostable/1
  E_mJ/1 -> gain/1
  Monostable/1 -> Switch1/2
  Constant2/1 -> Switch1/1
  Constant3/1 -> Switch1/3
  Switch1/1 -> Product1/2

== system transfer_function_calculation/Generator/3 Level Converter2/Loss Calculation/Leg B1/Subsystem/Loss Calculation Unit/Demux IGBTs and Diodes Currents and voltages/Subsystem1 ==
  I : Inport
  Gain1 : Gain  Gain=-1
  Saturation2 : Saturate  UpperLimit=1e6  LowerLimit=0
  Saturation3 : Saturate  UpperLimit=0  LowerLimit=-1e6
  I_Q : Outport
  I_D : Outport  Port=2
  wires:
  Gain1/1 -> I_D/1
  Saturation2/1 -> I_Q/1
  I/1 -> Saturation3/1, Saturation2/1
  Saturation3/1 -> Gain1/1

== system transfer_function_calculation/Generator/3 Level Converter2/Loss Calculation/Leg B1/Subsystem/Loss Calculation Unit/Demux IGBTs and Diodes Currents and voltages/Subsystem2 ==
  I : Inport
  Gain1 : Gain  Gain=-1
  Saturation2 : Saturate  UpperLimit=1e6  LowerLimit=0
  Saturation3 : Saturate  UpperLimit=0  LowerLimit=-1e6
  I_Q : Outport
  I_D : Outport  Port=2
  wires:
  Saturation3/1 -> Gain1/1
  I/1 -> Saturation2/1, Saturation3/1
  Saturation2/1 -> I_Q/1
  Gain1/1 -> I_D/1

== system transfer_function_calculation/Generator/3 Level Converter2/Loss Calculation/Leg B1/Subsystem/Loss Calculation Unit/Diodes Losses Calculation/Energy-to-Power 2 ==
  Trig : Inport
  E_mJ : Inport  Port=2
  Constant2 : Constant
  Constant3 : Constant  Value=0
  Monostable : powerlib_meascontrol/Logic/Monostable  EdgeDetect=Rising  PulseDuration=ceil(PulseDuration/Ts)*Ts  ic=0  Ts=Ts
  Product1 : Product  RndMeth=Zero
  Sample and Hold : powerlib_meascontrol/Additional Components/Sample and Hold  ic=0  Ts=Ts
  Switch1 : Switch  Criteria=u2 ~= 0
  gain : Gain  Gain=1e-3/(ceil(PulseDuration/Ts)*Ts)
  P_W : Outport
  wires:
  Switch1/1 -> Product1/2
  Constant3/1 -> Switch1/3
  Constant2/1 -> Switch1/1
  Monostable/1 -> Switch1/2
  E_mJ/1 -> gain/1
  Trig/1 -> Monostable/1, Sample and Hold/2
  gain/1 -> Sample and Hold/1
  Sample and Hold/1 -> Product1/1
  Product1/1 -> P_W/1

== system transfer_function_calculation/Generator/3 Level Converter2/Loss Calculation/Leg B1/Subsystem/Loss Calculation Unit/IGBTs Losses Calculation/Energy-to-Power 1 ==
  Trig : Inport
  E_mJ : Inport  Port=2
  Constant2 : Constant
  Constant3 : Constant  Value=0
  Monostable : powerlib_meascontrol/Logic/Monostable  EdgeDetect=Rising  PulseDuration=ceil(PulseDuration/Ts)*Ts  ic=0  Ts=Ts
  Product1 : Product  RndMeth=Zero
  Sample and Hold : powerlib_meascontrol/Additional Components/Sample and Hold  ic=0  Ts=Ts
  Switch1 : Switch  Criteria=u2 ~= 0
  gain : Gain  Gain=1e-3/(ceil(PulseDuration/Ts)*Ts)
  P_W : Outport
  wires:
  Switch1/1 -> Product1/2
  Constant3/1 -> Switch1/3
  Constant2/1 -> Switch1/1
  Monostable/1 -> Switch1/2
  E_mJ/1 -> gain/1
  Trig/1 -> Monostable/1, Sample and Hold/2
  gain/1 -> Sample and Hold/1
  Sample and Hold/1 -> Product1/1
  Product1/1 -> P_W/1

== system transfer_function_calculation/Generator/3 Level Converter2/Loss Calculation/Leg B1/Subsystem/Loss Calculation Unit/IGBTs Losses Calculation/Energy-to-Power 2 ==
  Trig : Inport
  E_mJ : Inport  Port=2
  Constant2 : Constant
  Constant3 : Constant  Value=0
  Monostable : powerlib_meascontrol/Logic/Monostable  EdgeDetect=Rising  PulseDuration=ceil(PulseDuration/Ts)*Ts  ic=0  Ts=Ts
  Product1 : Product  RndMeth=Zero
  Sample and Hold : powerlib_meascontrol/Additional Components/Sample and Hold  ic=0  Ts=Ts
  Switch1 : Switch  Criteria=u2 ~= 0
  gain : Gain  Gain=1e-3/(ceil(PulseDuration/Ts)*Ts)
  P_W : Outport
  wires:
  Switch1/1 -> Product1/2
  Constant3/1 -> Switch1/3
  Constant2/1 -> Switch1/1
  Monostable/1 -> Switch1/2
  E_mJ/1 -> gain/1
  Trig/1 -> Monostable/1, Sample and Hold/2
  gain/1 -> Sample and Hold/1
  Sample and Hold/1 -> Product1/1
  Product1/1 -> P_W/1

== system transfer_function_calculation/Generator/3 Level Converter2/Loss Calculation/Leg B2/Subsystem/Loss Calculation Unit/Demux IGBTs and Diodes Currents and voltages/Subsystem1 ==
  I : Inport
  Gain1 : Gain  Gain=-1
  Saturation2 : Saturate  UpperLimit=1e6  LowerLimit=0
  Saturation3 : Saturate  UpperLimit=0  LowerLimit=-1e6
  I_Q : Outport
  I_D : Outport  Port=2
  wires:
  Saturation3/1 -> Gain1/1
  I/1 -> Saturation2/1, Saturation3/1
  Saturation2/1 -> I_Q/1
  Gain1/1 -> I_D/1

== system transfer_function_calculation/Generator/3 Level Converter2/Loss Calculation/Leg B2/Subsystem/Loss Calculation Unit/Demux IGBTs and Diodes Currents and voltages/Subsystem2 ==
  I : Inport
  Gain1 : Gain  Gain=-1
  Saturation2 : Saturate  UpperLimit=1e6  LowerLimit=0
  Saturation3 : Saturate  UpperLimit=0  LowerLimit=-1e6
  I_Q : Outport
  I_D : Outport  Port=2
  wires:
  Gain1/1 -> I_D/1
  Saturation2/1 -> I_Q/1
  I/1 -> Saturation3/1, Saturation2/1
  Saturation3/1 -> Gain1/1

== system transfer_function_calculation/Generator/3 Level Converter2/Loss Calculation/Leg B2/Subsystem/Loss Calculation Unit/Diodes Losses Calculation/Energy-to-Power 2 ==
  Trig : Inport
  E_mJ : Inport  Port=2
  Constant2 : Constant
  Constant3 : Constant  Value=0
  Monostable : powerlib_meascontrol/Logic/Monostable  EdgeDetect=Rising  PulseDuration=ceil(PulseDuration/Ts)*Ts  ic=0  Ts=Ts
  Product1 : Product  RndMeth=Zero
  Sample and Hold : powerlib_meascontrol/Additional Components/Sample and Hold  ic=0  Ts=Ts
  Switch1 : Switch  Criteria=u2 ~= 0
  gain : Gain  Gain=1e-3/(ceil(PulseDuration/Ts)*Ts)
  P_W : Outport
  wires:
  Product1/1 -> P_W/1
  Sample and Hold/1 -> Product1/1
  gain/1 -> Sample and Hold/1
  Trig/1 -> Sample and Hold/2, Monostable/1
  E_mJ/1 -> gain/1
  Monostable/1 -> Switch1/2
  Constant2/1 -> Switch1/1
  Constant3/1 -> Switch1/3
  Switch1/1 -> Product1/2

== system transfer_function_calculation/Generator/3 Level Converter2/Loss Calculation/Leg B2/Subsystem/Loss Calculation Unit/IGBTs Losses Calculation/Energy-to-Power 1 ==
  Trig : Inport
  E_mJ : Inport  Port=2
  Constant2 : Constant
  Constant3 : Constant  Value=0
  Monostable : powerlib_meascontrol/Logic/Monostable  EdgeDetect=Rising  PulseDuration=ceil(PulseDuration/Ts)*Ts  ic=0  Ts=Ts
  Product1 : Product  RndMeth=Zero
  Sample and Hold : powerlib_meascontrol/Additional Components/Sample and Hold  ic=0  Ts=Ts
  Switch1 : Switch  Criteria=u2 ~= 0
  gain : Gain  Gain=1e-3/(ceil(PulseDuration/Ts)*Ts)
  P_W : Outport
  wires:
  Product1/1 -> P_W/1
  Sample and Hold/1 -> Product1/1
  gain/1 -> Sample and Hold/1
  Trig/1 -> Sample and Hold/2, Monostable/1
  E_mJ/1 -> gain/1
  Monostable/1 -> Switch1/2
  Constant2/1 -> Switch1/1
  Constant3/1 -> Switch1/3
  Switch1/1 -> Product1/2

== system transfer_function_calculation/Generator/3 Level Converter2/Loss Calculation/Leg B2/Subsystem/Loss Calculation Unit/IGBTs Losses Calculation/Energy-to-Power 2 ==
  Trig : Inport
  E_mJ : Inport  Port=2
  Constant2 : Constant
  Constant3 : Constant  Value=0
  Monostable : powerlib_meascontrol/Logic/Monostable  EdgeDetect=Rising  PulseDuration=ceil(PulseDuration/Ts)*Ts  ic=0  Ts=Ts
  Product1 : Product  RndMeth=Zero
  Sample and Hold : powerlib_meascontrol/Additional Components/Sample and Hold  ic=0  Ts=Ts
  Switch1 : Switch  Criteria=u2 ~= 0
  gain : Gain  Gain=1e-3/(ceil(PulseDuration/Ts)*Ts)
  P_W : Outport
  wires:
  Product1/1 -> P_W/1
  Sample and Hold/1 -> Product1/1
  gain/1 -> Sample and Hold/1
  Trig/1 -> Sample and Hold/2, Monostable/1
  E_mJ/1 -> gain/1
  Monostable/1 -> Switch1/2
  Constant2/1 -> Switch1/1
  Constant3/1 -> Switch1/3
  Switch1/1 -> Product1/2

== system transfer_function_calculation/Generator/3 Level Converter2/Loss Calculation/Leg C1/Subsystem/Loss Calculation Unit/Demux IGBTs and Diodes Currents and voltages/Subsystem1 ==
  I : Inport
  Gain1 : Gain  Gain=-1
  Saturation2 : Saturate  UpperLimit=1e6  LowerLimit=0
  Saturation3 : Saturate  UpperLimit=0  LowerLimit=-1e6
  I_Q : Outport
  I_D : Outport  Port=2
  wires:
  Gain1/1 -> I_D/1
  Saturation2/1 -> I_Q/1
  I/1 -> Saturation3/1, Saturation2/1
  Saturation3/1 -> Gain1/1

== system transfer_function_calculation/Generator/3 Level Converter2/Loss Calculation/Leg C1/Subsystem/Loss Calculation Unit/Demux IGBTs and Diodes Currents and voltages/Subsystem2 ==
  I : Inport
  Gain1 : Gain  Gain=-1
  Saturation2 : Saturate  UpperLimit=1e6  LowerLimit=0
  Saturation3 : Saturate  UpperLimit=0  LowerLimit=-1e6
  I_Q : Outport
  I_D : Outport  Port=2
  wires:
  Saturation3/1 -> Gain1/1
  I/1 -> Saturation2/1, Saturation3/1
  Saturation2/1 -> I_Q/1
  Gain1/1 -> I_D/1

== system transfer_function_calculation/Generator/3 Level Converter2/Loss Calculation/Leg C1/Subsystem/Loss Calculation Unit/Diodes Losses Calculation/Energy-to-Power 2 ==
  Trig : Inport
  E_mJ : Inport  Port=2
  Constant2 : Constant
  Constant3 : Constant  Value=0
  Monostable : powerlib_meascontrol/Logic/Monostable  EdgeDetect=Rising  PulseDuration=ceil(PulseDuration/Ts)*Ts  ic=0  Ts=Ts
  Product1 : Product  RndMeth=Zero
  Sample and Hold : powerlib_meascontrol/Additional Components/Sample and Hold  ic=0  Ts=Ts
  Switch1 : Switch  Criteria=u2 ~= 0
  gain : Gain  Gain=1e-3/(ceil(PulseDuration/Ts)*Ts)
  P_W : Outport
  wires:
  Switch1/1 -> Product1/2
  Constant3/1 -> Switch1/3
  Constant2/1 -> Switch1/1
  Monostable/1 -> Switch1/2
  E_mJ/1 -> gain/1
  Trig/1 -> Monostable/1, Sample and Hold/2
  gain/1 -> Sample and Hold/1
  Sample and Hold/1 -> Product1/1
  Product1/1 -> P_W/1

== system transfer_function_calculation/Generator/3 Level Converter2/Loss Calculation/Leg C1/Subsystem/Loss Calculation Unit/IGBTs Losses Calculation/Energy-to-Power 1 ==
  Trig : Inport
  E_mJ : Inport  Port=2
  Constant2 : Constant
  Constant3 : Constant  Value=0
  Monostable : powerlib_meascontrol/Logic/Monostable  EdgeDetect=Rising  PulseDuration=ceil(PulseDuration/Ts)*Ts  ic=0  Ts=Ts
  Product1 : Product  RndMeth=Zero
  Sample and Hold : powerlib_meascontrol/Additional Components/Sample and Hold  ic=0  Ts=Ts
  Switch1 : Switch  Criteria=u2 ~= 0
  gain : Gain  Gain=1e-3/(ceil(PulseDuration/Ts)*Ts)
  P_W : Outport
  wires:
  Switch1/1 -> Product1/2
  Constant3/1 -> Switch1/3
  Constant2/1 -> Switch1/1
  Monostable/1 -> Switch1/2
  E_mJ/1 -> gain/1
  Trig/1 -> Monostable/1, Sample and Hold/2
  gain/1 -> Sample and Hold/1
  Sample and Hold/1 -> Product1/1
  Product1/1 -> P_W/1

== system transfer_function_calculation/Generator/3 Level Converter2/Loss Calculation/Leg C1/Subsystem/Loss Calculation Unit/IGBTs Losses Calculation/Energy-to-Power 2 ==
  Trig : Inport
  E_mJ : Inport  Port=2
  Constant2 : Constant
  Constant3 : Constant  Value=0
  Monostable : powerlib_meascontrol/Logic/Monostable  EdgeDetect=Rising  PulseDuration=ceil(PulseDuration/Ts)*Ts  ic=0  Ts=Ts
  Product1 : Product  RndMeth=Zero
  Sample and Hold : powerlib_meascontrol/Additional Components/Sample and Hold  ic=0  Ts=Ts
  Switch1 : Switch  Criteria=u2 ~= 0
  gain : Gain  Gain=1e-3/(ceil(PulseDuration/Ts)*Ts)
  P_W : Outport
  wires:
  Switch1/1 -> Product1/2
  Constant3/1 -> Switch1/3
  Constant2/1 -> Switch1/1
  Monostable/1 -> Switch1/2
  E_mJ/1 -> gain/1
  Trig/1 -> Monostable/1, Sample and Hold/2
  gain/1 -> Sample and Hold/1
  Sample and Hold/1 -> Product1/1
  Product1/1 -> P_W/1

== system transfer_function_calculation/Generator/3 Level Converter2/Loss Calculation/Leg C2/Subsystem/Loss Calculation Unit/Demux IGBTs and Diodes Currents and voltages/Subsystem1 ==
  I : Inport
  Gain1 : Gain  Gain=-1
  Saturation2 : Saturate  UpperLimit=1e6  LowerLimit=0
  Saturation3 : Saturate  UpperLimit=0  LowerLimit=-1e6
  I_Q : Outport
  I_D : Outport  Port=2
  wires:
  Saturation3/1 -> Gain1/1
  I/1 -> Saturation2/1, Saturation3/1
  Saturation2/1 -> I_Q/1
  Gain1/1 -> I_D/1

== system transfer_function_calculation/Generator/3 Level Converter2/Loss Calculation/Leg C2/Subsystem/Loss Calculation Unit/Demux IGBTs and Diodes Currents and voltages/Subsystem2 ==
  I : Inport
  Gain1 : Gain  Gain=-1
  Saturation2 : Saturate  UpperLimit=1e6  LowerLimit=0
  Saturation3 : Saturate  UpperLimit=0  LowerLimit=-1e6
  I_Q : Outport
  I_D : Outport  Port=2
  wires:
  Gain1/1 -> I_D/1
  Saturation2/1 -> I_Q/1
  I/1 -> Saturation3/1, Saturation2/1
  Saturation3/1 -> Gain1/1

== system transfer_function_calculation/Generator/3 Level Converter2/Loss Calculation/Leg C2/Subsystem/Loss Calculation Unit/Diodes Losses Calculation/Energy-to-Power 2 ==
  Trig : Inport
  E_mJ : Inport  Port=2
  Constant2 : Constant
  Constant3 : Constant  Value=0
  Monostable : powerlib_meascontrol/Logic/Monostable  EdgeDetect=Rising  PulseDuration=ceil(PulseDuration/Ts)*Ts  ic=0  Ts=Ts
  Product1 : Product  RndMeth=Zero
  Sample and Hold : powerlib_meascontrol/Additional Components/Sample and Hold  ic=0  Ts=Ts
  Switch1 : Switch  Criteria=u2 ~= 0
  gain : Gain  Gain=1e-3/(ceil(PulseDuration/Ts)*Ts)
  P_W : Outport
  wires:
  Product1/1 -> P_W/1
  Sample and Hold/1 -> Product1/1
  gain/1 -> Sample and Hold/1
  Trig/1 -> Sample and Hold/2, Monostable/1
  E_mJ/1 -> gain/1
  Monostable/1 -> Switch1/2
  Constant2/1 -> Switch1/1
  Constant3/1 -> Switch1/3
  Switch1/1 -> Product1/2

== system transfer_function_calculation/Generator/3 Level Converter2/Loss Calculation/Leg C2/Subsystem/Loss Calculation Unit/IGBTs Losses Calculation/Energy-to-Power 1 ==
  Trig : Inport
  E_mJ : Inport  Port=2
  Constant2 : Constant
  Constant3 : Constant  Value=0
  Monostable : powerlib_meascontrol/Logic/Monostable  EdgeDetect=Rising  PulseDuration=ceil(PulseDuration/Ts)*Ts  ic=0  Ts=Ts
  Product1 : Product  RndMeth=Zero
  Sample and Hold : powerlib_meascontrol/Additional Components/Sample and Hold  ic=0  Ts=Ts
  Switch1 : Switch  Criteria=u2 ~= 0
  gain : Gain  Gain=1e-3/(ceil(PulseDuration/Ts)*Ts)
  P_W : Outport
  wires:
  Product1/1 -> P_W/1
  Sample and Hold/1 -> Product1/1
  gain/1 -> Sample and Hold/1
  Trig/1 -> Sample and Hold/2, Monostable/1
  E_mJ/1 -> gain/1
  Monostable/1 -> Switch1/2
  Constant2/1 -> Switch1/1
  Constant3/1 -> Switch1/3
  Switch1/1 -> Product1/2

== system transfer_function_calculation/Generator/3 Level Converter2/Loss Calculation/Leg C2/Subsystem/Loss Calculation Unit/IGBTs Losses Calculation/Energy-to-Power 2 ==
  Trig : Inport
  E_mJ : Inport  Port=2
  Constant2 : Constant
  Constant3 : Constant  Value=0
  Monostable : powerlib_meascontrol/Logic/Monostable  EdgeDetect=Rising  PulseDuration=ceil(PulseDuration/Ts)*Ts  ic=0  Ts=Ts
  Product1 : Product  RndMeth=Zero
  Sample and Hold : powerlib_meascontrol/Additional Components/Sample and Hold  ic=0  Ts=Ts
  Switch1 : Switch  Criteria=u2 ~= 0
  gain : Gain  Gain=1e-3/(ceil(PulseDuration/Ts)*Ts)
  P_W : Outport
  wires:
  Product1/1 -> P_W/1
  Sample and Hold/1 -> Product1/1
  gain/1 -> Sample and Hold/1
  Trig/1 -> Sample and Hold/2, Monostable/1
  E_mJ/1 -> gain/1
  Monostable/1 -> Switch1/2
  Constant2/1 -> Switch1/1
  Constant3/1 -> Switch1/3
  Switch1/1 -> Product1/2
